simulink library "MBDS_Subsystems"  (R2018b)
settings: Solver=ode45  StartTime=0.0  StopTime=10.0  RelTol=1e-3
libraries: KIBES_Signal x1429, MBDS_Modules x44, simulink x2
(part 3 of 15)

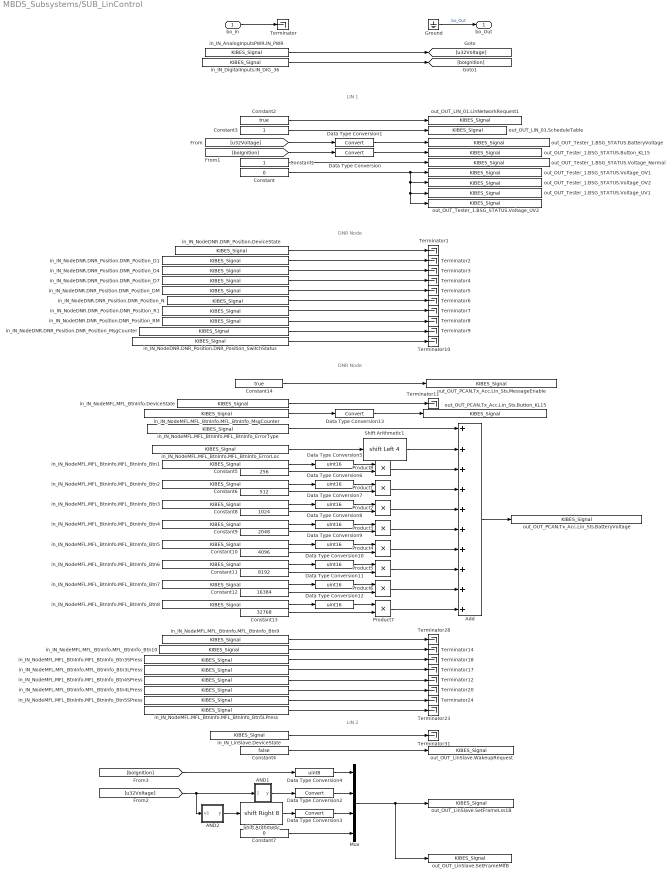
== system MBDS_Subsystems/SUB_LinControl ==
  note: LIN 2
  note: DNR Node
  note: DNR Node
  note: LIN 1
  bo_In : Inport  OutDataTypeStr=boolean
  AND1 : Subsystem  InitFcn=|  mask(AND){MBDS_LibraryBlock=on, BitwiseMode=on, Inputs=1, UseBitMask=on, BitMask='FF', OutDataTypeStr=Inherit: Inherit via back propagation, MBDS_BlockVersion=08.20.02}
      | if(exist('MBDS_BlockCallback', 'file'))
      |    MBDS_BlockCallback('Update', gcb);
      | end
      mask prompts: MBDS_LibraryBlock "MBDS library block"; BitwiseMode "Use 'bitwise' mode"; Inputs "Number of input ports:"; UseBitMask "Use bit mask"; BitMask "Bit mask:"; OutDataTypeStr "Output data type:"; MBDS_BlockVersion "Version:"
      mask help: Logical or bitwise AND operator. For multiple inputs, operators are applied across the inputs. For a single input, operators are applied across the input vector. In bitwise mode a bit mask can be applied onto single input signals.
      mask init: same as MBDS_Subsystems/SUB_DateTime/AND
      settings: AttributesFormatString=bitwise
      mask Help: eval(['open([workdir(''library_dir:''),''\Blockset\help\'',get_param(gcb,''MaskType''),''.html''])'])
      mask Callback BitwiseMode:
      | if(exist('MBDS_BlockCallback', 'file'))
      |    MBDS_BlockCallback('BitwiseMode', gcb);
      | end
      mask Callback Inputs:
      | if(exist('MBDS_BlockCallback', 'file'))
      |    MBDS_BlockCallback('Inputs', gcb);
      | end
      mask Callback UseBitMask:
      | if(exist('MBDS_BlockCallback', 'file'))
      |    MBDS_BlockCallback('UseBitMask', gcb);
      | end
      mask Callback BitMask:
      | if(exist('MBDS_BlockCallback', 'file'))
      |    MBDS_BlockCallback('BitMask', gcb);
      | end
      mask TypeOptions OutDataTypeStr: Inherit: Inherit via back propagation | int8 | uint8 | int16 | uint16 | int32 | uint32 | boolean
      mask Callback OutDataTypeStr:
      | % Adopt Value
      | if(exist('MBDS_BlockCallback', 'file'))
      |    MBDS_BlockCallback('OutDataTypeStr', gcb);
      | end
      mask DialogControl ParameterTabVar0 Prompt: Main
      mask DialogControl ParameterTabVar01 Prompt: Signal Attributes
      mask DialogControl ParameterTabVar012 Prompt: Version
      mask Display:
      | % Show icon or block text
      | if(UseBitMask)
      |    if(isnumeric(BitMask))
      |       BitMaskString = ['0x',dec2hex(floor(BitMask))];
      |    elseif(ischar(BitMask))
      |       BitMaskString = ['0x',upper(BitMask)];
      |    else
      |       BitMaskString = '???';
      |    end
      |    disp(sprintf(['AND\n', BitMaskString]))
      | else
      |    disp('AND')
      | end
  AND2 : Subsystem  InitFcn=|  mask(AND){MBDS_LibraryBlock=on, BitwiseMode=on, Inputs=1, UseBitMask=on, BitMask='FF00', OutDataTypeStr=Inherit: Inherit via back propagation, MBDS_BlockVersion=08.20.02}
      | if(exist('MBDS_BlockCallback', 'file'))
      |    MBDS_BlockCallback('Update', gcb);
      | end
      mask prompts: MBDS_LibraryBlock "MBDS library block"; BitwiseMode "Use 'bitwise' mode"; Inputs "Number of input ports:"; UseBitMask "Use bit mask"; BitMask "Bit mask:"; OutDataTypeStr "Output data type:"; MBDS_BlockVersion "Version:"
      mask help: Logical or bitwise AND operator. For multiple inputs, operators are applied across the inputs. For a single input, operators are applied across the input vector. In bitwise mode a bit mask can be applied onto single input signals.
      mask init: same as MBDS_Subsystems/SUB_DateTime/AND
      settings: AttributesFormatString=bitwise
      mask Help: eval(['open([workdir(''library_dir:''),''\Blockset\help\'',get_param(gcb,''MaskType''),''.html''])'])
      mask Callback BitwiseMode:
      | if(exist('MBDS_BlockCallback', 'file'))
      |    MBDS_BlockCallback('BitwiseMode', gcb);
      | end
      mask Callback Inputs:
      | if(exist('MBDS_BlockCallback', 'file'))
      |    MBDS_BlockCallback('Inputs', gcb);
      | end
      mask Callback UseBitMask:
      | if(exist('MBDS_BlockCallback', 'file'))
      |    MBDS_BlockCallback('UseBitMask', gcb);
      | end
      mask Callback BitMask:
      | if(exist('MBDS_BlockCallback', 'file'))
      |    MBDS_BlockCallback('BitMask', gcb);
      | end
      mask TypeOptions OutDataTypeStr: Inherit: Inherit via back propagation | int8 | uint8 | int16 | uint16 | int32 | uint32 | boolean
      mask Callback OutDataTypeStr:
      | % Adopt Value
      | if(exist('MBDS_BlockCallback', 'file'))
      |    MBDS_BlockCallback('OutDataTypeStr', gcb);
      | end
      mask DialogControl ParameterTabVar0 Prompt: Main
      mask DialogControl ParameterTabVar01 Prompt: Signal Attributes
      mask DialogControl ParameterTabVar012 Prompt: Version
      mask Display:
      | % Show icon or block text
      | if(UseBitMask)
      |    if(isnumeric(BitMask))
      |       BitMaskString = ['0x',dec2hex(floor(BitMask))];
      |    elseif(ischar(BitMask))
      |       BitMaskString = ['0x',upper(BitMask)];
      |    else
      |       BitMaskString = '???';
      |    end
      |    disp(sprintf(['AND\n', BitMaskString]))
      | else
      |    disp('AND')
      | end
  Add : Sum  InitFcn=|  Inputs=++++++++++  AccumDataTypeStr=uint16  OutDataTypeStr=uint16  SaturateOnIntegerOverflow=on
      | if(exist('MBDS_BlockCallback', 'file'))
      |    MBDS_BlockCallback('Update', gcb);  
      | end
      settings: AttributesFormatString=Saturate: %<SaturateOnIntegerOverflow>
  Constant : Constant  InitFcn=|  Value=0  OutDataTypeStr=uint8
      | if(exist('MBDS_BlockCallback', 'file'))
      |    MBDS_BlockCallback('Update', gcb);  
      | end
  Constant1 : Constant  InitFcn=|  OutDataTypeStr=uint8
      | if(exist('MBDS_BlockCallback', 'file'))
      |    MBDS_BlockCallback('Update', gcb);  
      | end
  Constant10 : Constant  InitFcn=|  Value=4096  OutDataTypeStr=uint16
      | if(exist('MBDS_BlockCallback', 'file'))
      |    MBDS_BlockCallback('Update', gcb);  
      | end
  Constant11 : Constant  InitFcn=|  Value=8192  OutDataTypeStr=uint16
      | if(exist('MBDS_BlockCallback', 'file'))
      |    MBDS_BlockCallback('Update', gcb);  
      | end
  Constant12 : Constant  InitFcn=|  Value=16384  OutDataTypeStr=uint16
      | if(exist('MBDS_BlockCallback', 'file'))
      |    MBDS_BlockCallback('Update', gcb);  
      | end
  Constant13 : Constant  InitFcn=|  Value=32768  OutDataTypeStr=uint16
      | if(exist('MBDS_BlockCallback', 'file'))
      |    MBDS_BlockCallback('Update', gcb);  
      | end
  Constant14 : Constant  InitFcn=|  Value=true  OutDataTypeStr=boolean  LockScale=on
      | if(exist('MBDS_BlockCallback', 'file'))
      |    MBDS_BlockCallback('Update', gcb);  
      | end
  Constant2 : Constant  InitFcn=|  Value=true  OutDataTypeStr=boolean
      | if(exist('MBDS_BlockCallback', 'file'))
      |    MBDS_BlockCallback('Update', gcb);  
      | end
  Constant3 : Constant  InitFcn=|  OutDataTypeStr=uint8
      | if(exist('MBDS_BlockCallback', 'file'))
      |    MBDS_BlockCallback('Update', gcb);  
      | end
  Constant4 : Constant  InitFcn=|  Value=false  OutDataTypeStr=boolean
      | if(exist('MBDS_BlockCallback', 'file'))
      |    MBDS_BlockCallback('Update', gcb);  
      | end
  Constant5 : Constant  InitFcn=|  Value=256  OutDataTypeStr=uint16
      | if(exist('MBDS_BlockCallback', 'file'))
      |    MBDS_BlockCallback('Update', gcb);  
      | end
  Constant6 : Constant  InitFcn=|  Value=512  OutDataTypeStr=uint16
      | if(exist('MBDS_BlockCallback', 'file'))
      |    MBDS_BlockCallback('Update', gcb);  
      | end
  Constant7 : Constant  InitFcn=|  Value=0  OutDataTypeStr=uint8
      | if(exist('MBDS_BlockCallback', 'file'))
      |    MBDS_BlockCallback('Update', gcb);  
      | end
  Constant8 : Constant  InitFcn=|  Value=1024  OutDataTypeStr=uint16
      | if(exist('MBDS_BlockCallback', 'file'))
      |    MBDS_BlockCallback('Update', gcb);  
      | end
  Constant9 : Constant  InitFcn=|  Value=2048  OutDataTypeStr=uint16
      | if(exist('MBDS_BlockCallback', 'file'))
      |    MBDS_BlockCallback('Update', gcb);  
      | end
  Data Type Conversion : DataTypeConversion  InitFcn=|  SaturateOnIntegerOverflow=on
      | try
      |    MBDS_BlockCallback('Update', gcb);
      | end
      settings: AttributesFormatString=Saturate: %<SaturateOnIntegerOverflow>
  Data Type Conversion1 : DataTypeConversion  InitFcn=|  SaturateOnIntegerOverflow=on
      | try
      |    MBDS_BlockCallback('Update', gcb);
      | end
      settings: AttributesFormatString=Saturate: %<SaturateOnIntegerOverflow>
  Data Type Conversion10 : DataTypeConversion  InitFcn=|  OutDataTypeStr=uint16  SaturateOnIntegerOverflow=on
      | try
      |    MBDS_BlockCallback('Update', gcb);
      | end
      settings: AttributesFormatString=Saturate: %<SaturateOnIntegerOverflow>
  Data Type Conversion11 : DataTypeConversion  InitFcn=|  OutDataTypeStr=uint16  SaturateOnIntegerOverflow=on
      | try
      |    MBDS_BlockCallback('Update', gcb);
      | end
      settings: AttributesFormatString=Saturate: %<SaturateOnIntegerOverflow>
  Data Type Conversion12 : DataTypeConversion  InitFcn=|  OutDataTypeStr=uint16  SaturateOnIntegerOverflow=on
      | try
      |    MBDS_BlockCallback('Update', gcb);
      | end
      settings: AttributesFormatString=Saturate: %<SaturateOnIntegerOverflow>
  Data Type Conversion13 : DataTypeConversion  InitFcn=|  SaturateOnIntegerOverflow=on
      | try
      |    MBDS_BlockCallback('Update', gcb);
      | end
      settings: AttributesFormatString=Saturate: %<SaturateOnIntegerOverflow>
  Data Type Conversion2 : DataTypeConversion  InitFcn=|
      | try
      |    MBDS_BlockCallback('Update', gcb);
      | end
      settings: AttributesFormatString=Saturate: %<SaturateOnIntegerOverflow>
  Data Type Conversion3 : DataTypeConversion  InitFcn=|
      | try
      |    MBDS_BlockCallback('Update', gcb);
      | end
      settings: AttributesFormatString=Saturate: %<SaturateOnIntegerOverflow>
  Data Type Conversion4 : DataTypeConversion  InitFcn=|  OutDataTypeStr=uint8  SaturateOnIntegerOverflow=on
      | try
      |    MBDS_BlockCallback('Update', gcb);
      | end
      settings: AttributesFormatString=Saturate: %<SaturateOnIntegerOverflow>
  Data Type Conversion5 : DataTypeConversion  InitFcn=|  OutDataTypeStr=uint16  SaturateOnIntegerOverflow=on
      | try
      |    MBDS_BlockCallback('Update', gcb);
      | end
      settings: AttributesFormatString=Saturate: %<SaturateOnIntegerOverflow>
  Data Type Conversion6 : DataTypeConversion  InitFcn=|  OutDataTypeStr=uint16  SaturateOnIntegerOverflow=on
      | try
      |    MBDS_BlockCallback('Update', gcb);
      | end
      settings: AttributesFormatString=Saturate: %<SaturateOnIntegerOverflow>
  Data Type Conversion7 : DataTypeConversion  InitFcn=|  OutDataTypeStr=uint16  SaturateOnIntegerOverflow=on
      | try
      |    MBDS_BlockCallback('Update', gcb);
      | end
      settings: AttributesFormatString=Saturate: %<SaturateOnIntegerOverflow>
  Data Type Conversion8 : DataTypeConversion  InitFcn=|  OutDataTypeStr=uint16  SaturateOnIntegerOverflow=on
      | try
      |    MBDS_BlockCallback('Update', gcb);
      | end
      settings: AttributesFormatString=Saturate: %<SaturateOnIntegerOverflow>
  Data Type Conversion9 : DataTypeConversion  InitFcn=|  OutDataTypeStr=uint16  SaturateOnIntegerOverflow=on
      | try
      |    MBDS_BlockCallback('Update', gcb);
      | end
      settings: AttributesFormatString=Saturate: %<SaturateOnIntegerOverflow>
  Ground : Ground  InitFcn=|
      | try
      |    MBDS_BlockCallback('Update', gcb);
      | end
      settings: MoveFcn=UpdateBlockSize(gcb);
  Mux : Mux  InitFcn=|
      | try
      |    MBDS_BlockCallback('Update', gcb);
      | end
  Product1 : Product  InitFcn=|  Inputs=**  OutDataTypeStr=uint16  SaturateOnIntegerOverflow=on
      | if(exist('MBDS_BlockCallback', 'file'))
      |    MBDS_BlockCallback('Update', gcb);  
      | end
      settings: AttributesFormatString=Saturate: %<SaturateOnIntegerOverflow>
  Product2 : Product  InitFcn=|  Inputs=**  OutDataTypeStr=uint16  SaturateOnIntegerOverflow=on
      | if(exist('MBDS_BlockCallback', 'file'))
      |    MBDS_BlockCallback('Update', gcb);  
      | end
      settings: AttributesFormatString=Saturate: %<SaturateOnIntegerOverflow>
  Product3 : Product  InitFcn=|  Inputs=**  OutDataTypeStr=uint16  SaturateOnIntegerOverflow=on
      | if(exist('MBDS_BlockCallback', 'file'))
      |    MBDS_BlockCallback('Update', gcb);  
      | end
      settings: AttributesFormatString=Saturate: %<SaturateOnIntegerOverflow>
  Product4 : Product  InitFcn=|  Inputs=**  OutDataTypeStr=uint16  SaturateOnIntegerOverflow=on
      | if(exist('MBDS_BlockCallback', 'file'))
      |    MBDS_BlockCallback('Update', gcb);  
      | end
      settings: AttributesFormatString=Saturate: %<SaturateOnIntegerOverflow>
  Product5 : Product  InitFcn=|  Inputs=**  OutDataTypeStr=uint16  SaturateOnIntegerOverflow=on
      | if(exist('MBDS_BlockCallback', 'file'))
      |    MBDS_BlockCallback('Update', gcb);  
      | end
      settings: AttributesFormatString=Saturate: %<SaturateOnIntegerOverflow>
  Product6 : Product  InitFcn=|  Inputs=**  OutDataTypeStr=uint16  SaturateOnIntegerOverflow=on
      | if(exist('MBDS_BlockCallback', 'file'))
      |    MBDS_BlockCallback('Update', gcb);  
      | end
      settings: AttributesFormatString=Saturate: %<SaturateOnIntegerOverflow>
  Product7 : Product  InitFcn=|  Inputs=**  OutDataTypeStr=uint16  SaturateOnIntegerOverflow=on
      | if(exist('MBDS_BlockCallback', 'file'))
      |    MBDS_BlockCallback('Update', gcb);  
      | end
      settings: AttributesFormatString=Saturate: %<SaturateOnIntegerOverflow>
  Product8 : Product  InitFcn=|  Inputs=**  OutDataTypeStr=uint16  SaturateOnIntegerOverflow=on
      | if(exist('MBDS_BlockCallback', 'file'))
      |    MBDS_BlockCallback('Update', gcb);  
      | end
      settings: AttributesFormatString=Saturate: %<SaturateOnIntegerOverflow>
  Shift Arithmetic : ArithShift  InitFcn=|  BitShiftNumber=8  BitShiftDirection=Right
      | try
      |    MBDS_BlockCallback('Update', gcb);
      | end
  Shift Arithmetic1 : ArithShift  InitFcn=|  BitShiftNumber=4  BitShiftDirection=Left
      | try
      |    MBDS_BlockCallback('Update', gcb);
      | end
  Terminator{,1..12,14,17..18,20,23..24,28,31} (21 alike) : Terminator
      settings: MoveFcn=UpdateBlockSize(gcb);
      settings: InitFcn=|
      | try
      |    MBDS_BlockCallback('Update', gcb);
      | end
  in_IN_AnalogInputsPWR.IN_PWR : KIBES_Signal/KIBES_Signal  MBDS_LibraryBlock=on  DatabaseKey=721  SignalName=IN_AnalogInputsPWR.IN_PWR  SymbolName=IN_AnalogInputsPWR_IN_PWR_000721  DataType=uint32  Init=0  Slope=1  Bias=0  DataSize=1  fpDataType=uint32  BlockIOType=Inport  DeviceType=0
  in_IN_DigitalInputs.IN_DIG_36 : KIBES_Signal/KIBES_Signal  MBDS_LibraryBlock=on  DatabaseKey=60  SignalName=IN_DigitalInputs.IN_DIG_36  SymbolName=IN_DigitalInputs_IN_DIG_36_000060  DataType=boolean  Init=0  Slope=1  Bias=0  DataSize=1  fpDataType=boolean  BlockIOType=Inport  DeviceType=0
  in_IN_LinSlave.DeviceState : KIBES_Signal/KIBES_Signal  MBDS_LibraryBlock=on  DatabaseKey=2325  SignalName=IN_LinSlave.DeviceState  SymbolName=IN_LinSlave_DeviceState_002325  DataType=uint16  Init=0  Slope=1  Bias=0  DataSize=1  fpDataType=uint16  BlockIOType=Inport  DeviceType=0
  in_IN_NodeDNR.DNR_Position.DNR_Position_D1 : KIBES_Signal/KIBES_Signal  MBDS_LibraryBlock=on  DatabaseKey=1352  SignalName=IN_NodeDNR.DNR_Position.DNR_Position_D1  SymbolName=IN_NodeDNR_DNR_Position_DNR_Position_D1_001352  DataType=uint8  Init=0  Slope=1  Bias=0  DataSize=1  fpDataType=uint8  BlockIOType=Inport  DeviceType=0
  in_IN_NodeDNR.DNR_Position.DNR_Position_D4 : KIBES_Signal/KIBES_Signal  MBDS_LibraryBlock=on  DatabaseKey=1353  SignalName=IN_NodeDNR.DNR_Position.DNR_Position_D4  SymbolName=IN_NodeDNR_DNR_Position_DNR_Position_D4_001353  DataType=uint8  Init=0  Slope=1  Bias=0  DataSize=1  fpDataType=uint8  BlockIOType=Inport  DeviceType=0
  in_IN_NodeDNR.DNR_Position.DNR_Position_D7 : KIBES_Signal/KIBES_Signal  MBDS_LibraryBlock=on  DatabaseKey=1354  SignalName=IN_NodeDNR.DNR_Position.DNR_Position_D7  SymbolName=IN_NodeDNR_DNR_Position_DNR_Position_D7_001354  DataType=uint8  Init=0  Slope=1  Bias=0  DataSize=1  fpDataType=uint8  BlockIOType=Inport  DeviceType=0
  in_IN_NodeDNR.DNR_Position.DNR_Position_DM : KIBES_Signal/KIBES_Signal  MBDS_LibraryBlock=on  DatabaseKey=1355  SignalName=IN_NodeDNR.DNR_Position.DNR_Position_DM  SymbolName=IN_NodeDNR_DNR_Position_DNR_Position_DM_001355  DataType=uint8  Init=0  Slope=1  Bias=0  DataSize=1  fpDataType=uint8  BlockIOType=Inport  DeviceType=0
  in_IN_NodeDNR.DNR_Position.DNR_Position_MsgCounter : KIBES_Signal/KIBES_Signal  MBDS_LibraryBlock=on  DatabaseKey=1356  SignalName=IN_NodeDNR.DNR_Position.DNR_Position_MsgCounter  SymbolName=IN_NodeDNR_DNR_Position_DNR_Position_MsgCounter_001356  DataType=uint8  Init=0  Slope=1  Bias=0  DataSize=1  fpDataType=uint8  BlockIOType=Inport  DeviceType=0
  in_IN_NodeDNR.DNR_Position.DNR_Position_N : KIBES_Signal/KIBES_Signal  MBDS_LibraryBlock=on  DatabaseKey=1351  SignalName=IN_NodeDNR.DNR_Position.DNR_Position_N  SymbolName=IN_NodeDNR_DNR_Position_DNR_Position_N_001351  DataType=uint8  Init=0  Slope=1  Bias=0  DataSize=1  fpDataType=uint8  BlockIOType=Inport  DeviceType=0
  in_IN_NodeDNR.DNR_Position.DNR_Position_R1 : KIBES_Signal/KIBES_Signal  MBDS_LibraryBlock=on  DatabaseKey=1350  SignalName=IN_NodeDNR.DNR_Position.DNR_Position_R1  SymbolName=IN_NodeDNR_DNR_Position_DNR_Position_R1_001350  DataType=uint8  Init=0  Slope=1  Bias=0  DataSize=1  fpDataType=uint8  BlockIOType=Inport  DeviceType=0
  in_IN_NodeDNR.DNR_Position.DNR_Position_RM : KIBES_Signal/KIBES_Signal  MBDS_LibraryBlock=on  DatabaseKey=1349  SignalName=IN_NodeDNR.DNR_Position.DNR_Position_RM  SymbolName=IN_NodeDNR_DNR_Position_DNR_Position_RM_001349  DataType=uint8  Init=0  Slope=1  Bias=0  DataSize=1  fpDataType=uint8  BlockIOType=Inport  DeviceType=0
  in_IN_NodeDNR.DNR_Position.DNR_Position_SwitchStatus : KIBES_Signal/KIBES_Signal  MBDS_LibraryBlock=on  DatabaseKey=1357  SignalName=IN_NodeDNR.DNR_Position.DNR_Position_SwitchStatus  SymbolName=IN_NodeDNR_DNR_Position_DNR_Position_SwitchStatus_001357  DataType=uint8  Init=0  Slope=1  Bias=0  DataSize=1  fpDataType=uint8  BlockIOType=Inport  DeviceType=0
  in_IN_NodeDNR.DNR_Position.DeviceState : KIBES_Signal/KIBES_Signal  MBDS_LibraryBlock=on  DatabaseKey=2273  SignalName=IN_NodeDNR.DNR_Position.DeviceState  SymbolName=IN_NodeDNR_DNR_Position_DeviceState_002273  DataType=uint16  Init=0  Slope=1  Bias=0  DataSize=1  fpDataType=uint16  BlockIOType=Inport  DeviceType=0
  in_IN_NodeMFL.MFL_BtnInfo.DeviceState : KIBES_Signal/KIBES_Signal  MBDS_LibraryBlock=on  DatabaseKey=2272  SignalName=IN_NodeMFL.MFL_BtnInfo.DeviceState  SymbolName=IN_NodeMFL_MFL_BtnInfo_DeviceState_002272  DataType=uint16  Init=0  Slope=1  Bias=0  DataSize=1  fpDataType=uint16  BlockIOType=Inport  DeviceType=0
  in_IN_NodeMFL.MFL_BtnInfo.MFL_BtnInfo_Btn1 : KIBES_Signal/KIBES_Signal  MBDS_LibraryBlock=on  DatabaseKey=1361  SignalName=IN_NodeMFL.MFL_BtnInfo.MFL_BtnInfo_Btn1  SymbolName=IN_NodeMFL_MFL_BtnInfo_MFL_BtnInfo_Btn1_001361  DataType=uint8  Init=0  Slope=1  Bias=0  DataSize=1  fpDataType=uint8  BlockIOType=Inport  DeviceType=0
  in_IN_NodeMFL.MFL_BtnInfo.MFL_BtnInfo_Btn10 : KIBES_Signal/KIBES_Signal  MBDS_LibraryBlock=on  DatabaseKey=1370  SignalName=IN_NodeMFL.MFL_BtnInfo.MFL_BtnInfo_Btn10  SymbolName=IN_NodeMFL_MFL_BtnInfo_MFL_BtnInfo_Btn10_001370  DataType=uint8  Init=0  Slope=1  Bias=0  DataSize=1  fpDataType=uint8  BlockIOType=Inport  DeviceType=0
  in_IN_NodeMFL.MFL_BtnInfo.MFL_BtnInfo_Btn2 : KIBES_Signal/KIBES_Signal  MBDS_LibraryBlock=on  DatabaseKey=1362  SignalName=IN_NodeMFL.MFL_BtnInfo.MFL_BtnInfo_Btn2  SymbolName=IN_NodeMFL_MFL_BtnInfo_MFL_BtnInfo_Btn2_001362  DataType=uint8  Init=0  Slope=1  Bias=0  DataSize=1  fpDataType=uint8  BlockIOType=Inport  DeviceType=0
  in_IN_NodeMFL.MFL_BtnInfo.MFL_BtnInfo_Btn3 : KIBES_Signal/KIBES_Signal  MBDS_LibraryBlock=on  DatabaseKey=1363  SignalName=IN_NodeMFL.MFL_BtnInfo.MFL_BtnInfo_Btn3  SymbolName=IN_NodeMFL_MFL_BtnInfo_MFL_BtnInfo_Btn3_001363  DataType=uint8  Init=0  Slope=1  Bias=0  DataSize=1  fpDataType=uint8  BlockIOType=Inport  DeviceType=0
  in_IN_NodeMFL.MFL_BtnInfo.MFL_BtnInfo_Btn3LPress : KIBES_Signal/KIBES_Signal  MBDS_LibraryBlock=on  DatabaseKey=1372  SignalName=IN_NodeMFL.MFL_BtnInfo.MFL_BtnInfo_Btn3LPress  SymbolName=IN_NodeMFL_MFL_BtnInfo_MFL_BtnInfo_Btn3LPress_001372  DataType=uint8  Init=0  Slope=1  Bias=0  DataSize=1  fpDataType=uint8  BlockIOType=Inport  DeviceType=0
  in_IN_NodeMFL.MFL_BtnInfo.MFL_BtnInfo_Btn3SPress : KIBES_Signal/KIBES_Signal  MBDS_LibraryBlock=on  DatabaseKey=1371  SignalName=IN_NodeMFL.MFL_BtnInfo.MFL_BtnInfo_Btn3SPress  SymbolName=IN_NodeMFL_MFL_BtnInfo_MFL_BtnInfo_Btn3SPress_001371  DataType=uint8  Init=0  Slope=1  Bias=0  DataSize=1  fpDataType=uint8  BlockIOType=Inport  DeviceType=0
  in_IN_NodeMFL.MFL_BtnInfo.MFL_BtnInfo_Btn4 : KIBES_Signal/KIBES_Signal  MBDS_LibraryBlock=on  DatabaseKey=1364  SignalName=IN_NodeMFL.MFL_BtnInfo.MFL_BtnInfo_Btn4  SymbolName=IN_NodeMFL_MFL_BtnInfo_MFL_BtnInfo_Btn4_001364  DataType=uint8  Init=0  Slope=1  Bias=0  DataSize=1  fpDataType=uint8  BlockIOType=Inport  DeviceType=0
  in_IN_NodeMFL.MFL_BtnInfo.MFL_BtnInfo_Btn4LPress : KIBES_Signal/KIBES_Signal  MBDS_LibraryBlock=on  DatabaseKey=1374  SignalName=IN_NodeMFL.MFL_BtnInfo.MFL_BtnInfo_Btn4LPress  SymbolName=IN_NodeMFL_MFL_BtnInfo_MFL_BtnInfo_Btn4LPress_001374  DataType=uint8  Init=0  Slope=1  Bias=0  DataSize=1  fpDataType=uint8  BlockIOType=Inport  DeviceType=0
  in_IN_NodeMFL.MFL_BtnInfo.MFL_BtnInfo_Btn4SPress : KIBES_Signal/KIBES_Signal  MBDS_LibraryBlock=on  DatabaseKey=1373  SignalName=IN_NodeMFL.MFL_BtnInfo.MFL_BtnInfo_Btn4SPress  SymbolName=IN_NodeMFL_MFL_BtnInfo_MFL_BtnInfo_Btn4SPress_001373  DataType=uint8  Init=0  Slope=1  Bias=0  DataSize=1  fpDataType=uint8  BlockIOType=Inport  DeviceType=0
  in_IN_NodeMFL.MFL_BtnInfo.MFL_BtnInfo_Btn5 : KIBES_Signal/KIBES_Signal  MBDS_LibraryBlock=on  DatabaseKey=1365  SignalName=IN_NodeMFL.MFL_BtnInfo.MFL_BtnInfo_Btn5  SymbolName=IN_NodeMFL_MFL_BtnInfo_MFL_BtnInfo_Btn5_001365  DataType=uint8  Init=0  Slope=1  Bias=0  DataSize=1  fpDataType=uint8  BlockIOType=Inport  DeviceType=0
  in_IN_NodeMFL.MFL_BtnInfo.MFL_BtnInfo_Btn5LPress : KIBES_Signal/KIBES_Signal  MBDS_LibraryBlock=on  DatabaseKey=1376  SignalName=IN_NodeMFL.MFL_BtnInfo.MFL_BtnInfo_Btn5LPress  SymbolName=IN_NodeMFL_MFL_BtnInfo_MFL_BtnInfo_Btn5LPress_001376  DataType=uint8  Init=0  Slope=1  Bias=0  DataSize=1  fpDataType=uint8  BlockIOType=Inport  DeviceType=0
  in_IN_NodeMFL.MFL_BtnInfo.MFL_BtnInfo_Btn5SPress : KIBES_Signal/KIBES_Signal  MBDS_LibraryBlock=on  DatabaseKey=1375  SignalName=IN_NodeMFL.MFL_BtnInfo.MFL_BtnInfo_Btn5SPress  SymbolName=IN_NodeMFL_MFL_BtnInfo_MFL_BtnInfo_Btn5SPress_001375  DataType=uint8  Init=0  Slope=1  Bias=0  DataSize=1  fpDataType=uint8  BlockIOType=Inport  DeviceType=0
  in_IN_NodeMFL.MFL_BtnInfo.MFL_BtnInfo_Btn6 : KIBES_Signal/KIBES_Signal  MBDS_LibraryBlock=on  DatabaseKey=1366  SignalName=IN_NodeMFL.MFL_BtnInfo.MFL_BtnInfo_Btn6  SymbolName=IN_NodeMFL_MFL_BtnInfo_MFL_BtnInfo_Btn6_001366  DataType=uint8  Init=0  Slope=1  Bias=0  DataSize=1  fpDataType=uint8  BlockIOType=Inport  DeviceType=0
  in_IN_NodeMFL.MFL_BtnInfo.MFL_BtnInfo_Btn7 : KIBES_Signal/KIBES_Signal  MBDS_LibraryBlock=on  DatabaseKey=1367  SignalName=IN_NodeMFL.MFL_BtnInfo.MFL_BtnInfo_Btn7  SymbolName=IN_NodeMFL_MFL_BtnInfo_MFL_BtnInfo_Btn7_001367  DataType=uint8  Init=0  Slope=1  Bias=0  DataSize=1  fpDataType=uint8  BlockIOType=Inport  DeviceType=0
  in_IN_NodeMFL.MFL_BtnInfo.MFL_BtnInfo_Btn8 : KIBES_Signal/KIBES_Signal  MBDS_LibraryBlock=on  DatabaseKey=1368  SignalName=IN_NodeMFL.MFL_BtnInfo.MFL_BtnInfo_Btn8  SymbolName=IN_NodeMFL_MFL_BtnInfo_MFL_BtnInfo_Btn8_001368  DataType=uint8  Init=0  Slope=1  Bias=0  DataSize=1  fpDataType=uint8  BlockIOType=Inport  DeviceType=0
  in_IN_NodeMFL.MFL_BtnInfo.MFL_BtnInfo_Btn9 : KIBES_Signal/KIBES_Signal  MBDS_LibraryBlock=on  DatabaseKey=1369  SignalName=IN_NodeMFL.MFL_BtnInfo.MFL_BtnInfo_Btn9  SymbolName=IN_NodeMFL_MFL_BtnInfo_MFL_BtnInfo_Btn9_001369  DataType=uint8  Init=0  Slope=1  Bias=0  DataSize=1  fpDataType=uint8  BlockIOType=Inport  DeviceType=0
  in_IN_NodeMFL.MFL_BtnInfo.MFL_BtnInfo_ErrorLoc : KIBES_Signal/KIBES_Signal  MBDS_LibraryBlock=on  DatabaseKey=1360  SignalName=IN_NodeMFL.MFL_BtnInfo.MFL_BtnInfo_ErrorLoc  SymbolName=IN_NodeMFL_MFL_BtnInfo_MFL_BtnInfo_ErrorLoc_001360  DataType=uint8  Init=0  Slope=1  Bias=0  DataSize=1  fpDataType=uint8  BlockIOType=Inport  DeviceType=0
  in_IN_NodeMFL.MFL_BtnInfo.MFL_BtnInfo_ErrorType : KIBES_Signal/KIBES_Signal  MBDS_LibraryBlock=on  DatabaseKey=1359  SignalName=IN_NodeMFL.MFL_BtnInfo.MFL_BtnInfo_ErrorType  SymbolName=IN_NodeMFL_MFL_BtnInfo_MFL_BtnInfo_ErrorType_001359  DataType=uint8  Init=0  Slope=1  Bias=0  DataSize=1  fpDataType=uint8  BlockIOType=Inport  DeviceType=0
  in_IN_NodeMFL.MFL_BtnInfo.MFL_BtnInfo_MsgCounter : KIBES_Signal/KIBES_Signal  MBDS_LibraryBlock=on  DatabaseKey=1358  SignalName=IN_NodeMFL.MFL_BtnInfo.MFL_BtnInfo_MsgCounter  SymbolName=IN_NodeMFL_MFL_BtnInfo_MFL_BtnInfo_MsgCounter_001358  DataType=uint8  Init=0  Slope=1  Bias=0  DataSize=1  fpDataType=uint8  BlockIOType=Inport  DeviceType=0
  out_OUT_LIN_01.LinNetworkRequest1 : KIBES_Signal/KIBES_Signal  MBDS_LibraryBlock=on  DatabaseKey=1396  SignalName=OUT_LIN_01.LinNetworkRequest1  SymbolName=OUT_LIN_01_LinNetworkRequest1_001396  DataType=boolean  Init=0  Slope=1  Bias=0  DataSize=1  fpDataType=boolean  BlockIOType=Outport  DeviceType=0
  out_OUT_LIN_01.ScheduleTable : KIBES_Signal/KIBES_Signal  MBDS_LibraryBlock=on  DatabaseKey=1397  SignalName=OUT_LIN_01.ScheduleTable  SymbolName=OUT_LIN_01_ScheduleTable_001397  DataType=uint8  Init=0  Slope=1  Bias=0  DataSize=1  fpDataType=uint8  BlockIOType=Outport  DeviceType=0
  out_OUT_LinSlave.SetFrameLss1B : KIBES_Signal/KIBES_Signal  MBDS_LibraryBlock=on  DatabaseKey=2326  SignalName=OUT_LinSlave.SetFrameLss1B  SymbolName=OUT_LinSlave_SetFrameLss1B_002326  DataType=uint8  Init=[0 0 0 0]  Slope=1  Bias=0  DataSize=4  fpDataType=uint8  BlockIOType=Outport  DeviceType=0
  out_OUT_LinSlave.SetFrameMlfB : KIBES_Signal/KIBES_Signal  MBDS_LibraryBlock=on  DatabaseKey=2327  SignalName=OUT_LinSlave.SetFrameMlfB  SymbolName=OUT_LinSlave_SetFrameMlfB_002327  DataType=uint8  Init=[0 0 0 0]  Slope=1  Bias=0  DataSize=4  fpDataType=uint8  BlockIOType=Outport  DeviceType=0
  out_OUT_LinSlave.WakeupRequest : KIBES_Signal/KIBES_Signal  MBDS_LibraryBlock=on  DatabaseKey=2328  SignalName=OUT_LinSlave.WakeupRequest  SymbolName=OUT_LinSlave_WakeupRequest_002328  DataType=boolean  Init=0  Slope=1  Bias=0  DataSize=1  fpDataType=boolean  BlockIOType=Outport  DeviceType=0
  out_OUT_PCAN.Tx_Acc.Lin_Sts.BatteryVoltage : KIBES_Signal/KIBES_Signal  MBDS_LibraryBlock=on  DatabaseKey=1647  SignalName=OUT_PCAN.Tx_Acc.Lin_Sts.BatteryVoltage  SymbolName=OUT_PCAN_Tx_Acc_Lin_Sts_BatteryVoltage_001647  DataType=uint16  Init=0  Slope=1  Bias=0  DataSize=1  fpDataType=uint16  BlockIOType=Outport  DeviceType=0
  out_OUT_PCAN.Tx_Acc.Lin_Sts.Button_KL15 : KIBES_Signal/KIBES_Signal  MBDS_LibraryBlock=on  DatabaseKey=1648  SignalName=OUT_PCAN.Tx_Acc.Lin_Sts.Button_KL15  SymbolName=OUT_PCAN_Tx_Acc_Lin_Sts_Button_KL15_001648  DataType=boolean  Init=0  Slope=1  Bias=0  DataSize=1  fpDataType=boolean  BlockIOType=Outport  DeviceType=0
  out_OUT_PCAN.Tx_Acc.Lin_Sts.MessageEnable : KIBES_Signal/KIBES_Signal  MBDS_LibraryBlock=on  DatabaseKey=1677  SignalName=OUT_PCAN.Tx_Acc.Lin_Sts.MessageEnable  SymbolName=OUT_PCAN_Tx_Acc_Lin_Sts_MessageEnable_001677  DataType=boolean  Init=0  Slope=1  Bias=0  DataSize=1  fpDataType=boolean  BlockIOType=Outport  DeviceType=0
  out_OUT_Tester_1.BSG_STATUS.BatteryVoltage : KIBES_Signal/KIBES_Signal  MBDS_LibraryBlock=on  DatabaseKey=1395  SignalName=OUT_Tester_1.BSG_STATUS.BatteryVoltage  SymbolName=OUT_Tester_1_BSG_STATUS_BatteryVoltage_001395  DataType=uint16  Init=0  Slope=1  Bias=0  DataSize=1  fpDataType=uint16  BlockIOType=Outport  DeviceType=0
  out_OUT_Tester_1.BSG_STATUS.Button_KL15 : KIBES_Signal/KIBES_Signal  MBDS_LibraryBlock=on  DatabaseKey=1389  SignalName=OUT_Tester_1.BSG_STATUS.Button_KL15  SymbolName=OUT_Tester_1_BSG_STATUS_Button_KL15_001389  DataType=uint8  Init=0  Slope=1  Bias=0  DataSize=1  fpDataType=uint8  BlockIOType=Outport  DeviceType=0
  out_OUT_Tester_1.BSG_STATUS.Voltage_Normal : KIBES_Signal/KIBES_Signal  MBDS_LibraryBlock=on  DatabaseKey=1390  SignalName=OUT_Tester_1.BSG_STATUS.Voltage_Normal  SymbolName=OUT_Tester_1_BSG_STATUS_Voltage_Normal_001390  DataType=uint8  Init=0  Slope=1  Bias=0  DataSize=1  fpDataType=uint8  BlockIOType=Outport  DeviceType=0
  out_OUT_Tester_1.BSG_STATUS.Voltage_OV1 : KIBES_Signal/KIBES_Signal  MBDS_LibraryBlock=on  DatabaseKey=1391  SignalName=OUT_Tester_1.BSG_STATUS.Voltage_OV1  SymbolName=OUT_Tester_1_BSG_STATUS_Voltage_OV1_001391  DataType=uint8  Init=0  Slope=1  Bias=0  DataSize=1  fpDataType=uint8  BlockIOType=Outport  DeviceType=0
  out_OUT_Tester_1.BSG_STATUS.Voltage_OV2 : KIBES_Signal/KIBES_Signal  MBDS_LibraryBlock=on  DatabaseKey=1392  SignalName=OUT_Tester_1.BSG_STATUS.Voltage_OV2  SymbolName=OUT_Tester_1_BSG_STATUS_Voltage_OV2_001392  DataType=uint8  Init=0  Slope=1  Bias=0  DataSize=1  fpDataType=uint8  BlockIOType=Outport  DeviceType=0
  out_OUT_Tester_1.BSG_STATUS.Voltage_UV1 : KIBES_Signal/KIBES_Signal  MBDS_LibraryBlock=on  DatabaseKey=1393  SignalName=OUT_Tester_1.BSG_STATUS.Voltage_UV1  SymbolName=OUT_Tester_1_BSG_STATUS_Voltage_UV1_001393  DataType=uint8  Init=0  Slope=1  Bias=0  DataSize=1  fpDataType=uint8  BlockIOType=Outport  DeviceType=0
  out_OUT_Tester_1.BSG_STATUS.Voltage_UV2 : KIBES_Signal/KIBES_Signal  MBDS_LibraryBlock=on  DatabaseKey=1394  SignalName=OUT_Tester_1.BSG_STATUS.Voltage_UV2  SymbolName=OUT_Tester_1_BSG_STATUS_Voltage_UV2_001394  DataType=uint8  Init=0  Slope=1  Bias=0  DataSize=1  fpDataType=uint8  BlockIOType=Outport  DeviceType=0
  bo_Out : Outport  OutDataTypeStr=boolean
  wires:
  Data Type Conversion13/1 -> out_OUT_PCAN.Tx_Acc.Lin_Sts.Button_KL15/1
  Constant14/1 -> out_OUT_PCAN.Tx_Acc.Lin_Sts.MessageEnable/1
  Add/1 -> out_OUT_PCAN.Tx_Acc.Lin_Sts.BatteryVoltage/1
  Constant13/1 -> Product7/2
  Constant12/1 -> Product6/2
  Constant11/1 -> Product5/2
  Constant10/1 -> Product4/2
  Constant9/1 -> Product3/2
  Constant8/1 -> Product2/2
  Constant6/1 -> Product1/2
  Constant5/1 -> Product8/2
  Data Type Conversion12/1 -> Product7/1
  Data Type Conversion11/1 -> Product6/1
  Data Type Conversion10/1 -> Product5/1
  Data Type Conversion9/1 -> Product4/1
  Data Type Conversion8/1 -> Product3/1
  Data Type Conversion7/1 -> Product2/1
  Data Type Conversion6/1 -> Product1/1
  Data Type Conversion5/1 -> Product8/1
  Product7/1 -> Add/10
  Product6/1 -> Add/9
  Product5/1 -> Add/8
  Product4/1 -> Add/7
  Product3/1 -> Add/6
  Product2/1 -> Add/5
  Product1/1 -> Add/4
  Product8/1 -> Add/3
  Shift Arithmetic1/1 -> Add/2
  [boIgnition] -> Data Type Conversion4/1
  Data Type Conversion4/1 -> Mux/1
  Shift Arithmetic/1 -> Data Type Conversion3/1
  AND2/1(y) -> Shift Arithmetic/1
  Data Type Conversion3/1 -> Mux/3
  [u32Voltage] -> AND1/1(u1), AND2/1(u1)
  AND1/1(y) -> Data Type Conversion2/1
  Data Type Conversion2/1 -> Mux/2
  in_IN_DigitalInputs.IN_DIG_36/1 -> [boIgnition]
  in_IN_AnalogInputsPWR.IN_PWR/1 -> [u32Voltage]
  Constant7/1 -> Mux/4
  Mux/1 -> out_OUT_LinSlave.SetFrameLss1B/1, out_OUT_LinSlave.SetFrameMlfB/1
  Constant4/1 -> out_OUT_LinSlave.WakeupRequest/1
  in_IN_LinSlave.DeviceState/1 -> Terminator31/1
  in_IN_NodeMFL.MFL_BtnInfo.MFL_BtnInfo_MsgCounter/1 -> Data Type Conversion13/1
  in_IN_NodeMFL.MFL_BtnInfo.MFL_BtnInfo_ErrorType/1 -> Add/1
  in_IN_NodeMFL.MFL_BtnInfo.MFL_BtnInfo_ErrorLoc/1 -> Shift Arithmetic1/1
  in_IN_NodeMFL.MFL_BtnInfo.MFL_BtnInfo_Btn9/1 -> Terminator28/1
  in_IN_NodeMFL.MFL_BtnInfo.MFL_BtnInfo_Btn8/1 -> Data Type Conversion12/1
  in_IN_NodeMFL.MFL_BtnInfo.MFL_BtnInfo_Btn7/1 -> Data Type Conversion11/1
  in_IN_NodeMFL.MFL_BtnInfo.MFL_BtnInfo_Btn6/1 -> Data Type Conversion10/1
  in_IN_NodeMFL.MFL_BtnInfo.MFL_BtnInfo_Btn5SPress/1 -> Terminator24/1
  in_IN_NodeMFL.MFL_BtnInfo.MFL_BtnInfo_Btn5LPress/1 -> Terminator23/1
  in_IN_NodeMFL.MFL_BtnInfo.MFL_BtnInfo_Btn5/1 -> Data Type Conversion9/1
  in_IN_NodeMFL.MFL_BtnInfo.MFL_BtnInfo_Btn4SPress/1 -> Terminator12/1
  in_IN_NodeMFL.MFL_BtnInfo.MFL_BtnInfo_Btn4LPress/1 -> Terminator20/1
  in_IN_NodeMFL.MFL_BtnInfo.MFL_BtnInfo_Btn4/1 -> Data Type Conversion8/1
  in_IN_NodeMFL.MFL_BtnInfo.MFL_BtnInfo_Btn3SPress/1 -> Terminator18/1
  in_IN_NodeMFL.MFL_BtnInfo.MFL_BtnInfo_Btn3LPress/1 -> Terminator17/1
  in_IN_NodeMFL.MFL_BtnInfo.MFL_BtnInfo_Btn3/1 -> Data Type Conversion7/1
  in_IN_NodeMFL.MFL_BtnInfo.MFL_BtnInfo_Btn2/1 -> Data Type Conversion6/1
  in_IN_NodeMFL.MFL_BtnInfo.MFL_BtnInfo_Btn10/1 -> Terminator14/1
  in_IN_NodeMFL.MFL_BtnInfo.MFL_BtnInfo_Btn1/1 -> Data Type Conversion5/1
  in_IN_NodeMFL.MFL_BtnInfo.DeviceState/1 -> Terminator11/1
  in_IN_NodeDNR.DNR_Position.DNR_Position_SwitchStatus/1 -> Terminator10/1
  in_IN_NodeDNR.DNR_Position.DNR_Position_MsgCounter/1 -> Terminator9/1
  in_IN_NodeDNR.DNR_Position.DNR_Position_RM/1 -> Terminator8/1
  in_IN_NodeDNR.DNR_Position.DNR_Position_R1/1 -> Terminator7/1
  in_IN_NodeDNR.DNR_Position.DNR_Position_N/1 -> Terminator6/1
  in_IN_NodeDNR.DNR_Position.DNR_Position_DM/1 -> Terminator5/1
  in_IN_NodeDNR.DNR_Position.DNR_Position_D7/1 -> Terminator4/1
  in_IN_NodeDNR.DNR_Position.DNR_Position_D4/1 -> Terminator3/1
  in_IN_NodeDNR.DNR_Position.DNR_Position_D1/1 -> Terminator2/1
  in_IN_NodeDNR.DNR_Position.DeviceState/1 -> Terminator1/1
  Constant3/1 -> out_OUT_LIN_01.ScheduleTable/1
  Constant2/1 -> out_OUT_LIN_01.LinNetworkRequest1/1
  Data Type Conversion1/1 -> out_OUT_Tester_1.BSG_STATUS.BatteryVoltage/1
  [u32Voltage] -> Data Type Conversion1/1
  Data Type Conversion/1 -> out_OUT_Tester_1.BSG_STATUS.Button_KL15/1
  [boIgnition] -> Data Type Conversion/1
  Constant1/1 -> out_OUT_Tester_1.BSG_STATUS.Voltage_Normal/1
  Constant/1 -> out_OUT_Tester_1.BSG_STATUS.Voltage_OV1/1, out_OUT_Tester_1.BSG_STATUS.Voltage_OV2/1, out_OUT_Tester_1.BSG_STATUS.Voltage_UV1/1, out_OUT_Tester_1.BSG_STATUS.Voltage_UV2/1
  Ground/1 -> bo_Out/1  "bo_Out"
  bo_In/1 -> Terminator/1

== system MBDS_Subsystems/SUB_SystemStates ==
  note: After POR, force model hold equal true during WakeUpForceHoldTime
  note: Wake-up Inputs
  u16_WakeUpForceHoldTime : Inport  OutDataTypeStr=uint16
  Ground : Ground  InitFcn=|
      | try
      |    MBDS_BlockCallback('Update', gcb);
      | end
      settings: MoveFcn=UpdateBlockSize(gcb);
  ModelHoldForceTrue : Stateflow chart  TreatAsAtomicUnit=on
      settings: CopyFcn=|
      | if(exist('MBDS_BlockCallback', 'file'))
      |    MBDS_BlockCallback('Copy', gcb);
      | end
  NOT : Subsystem  InitFcn=|  mask(NOT){MBDS_LibraryBlock=on, BitwiseMode=off, Inputs=1, UseBitMask=off, BitMask='A1', OutDataTypeStr=Inherit: Inherit via back propagation, MBDS_BlockVersion=08.20.02}
      | if(exist('MBDS_BlockCallback', 'file'))
      |    MBDS_BlockCallback('Update', gcb);
      | end
      mask prompts: MBDS_LibraryBlock "MBDS library block"; BitwiseMode "Use 'bitwise' mode"; Inputs "Number of input ports:"; UseBitMask "Use bit mask"; BitMask "Bit mask:"; OutDataTypeStr "Output data type:"; MBDS_BlockVersion "Version:"
      mask help: Logical or bitwise NOT operator. The input value is inverted. In bitwise mode all bits of the input signal are inverted.
      mask init: same as MBDS_Subsystems/SUB_DateTime/AND
      mask Help: eval(['open([workdir(''library_dir:''),''\Blockset\help\'',get_param(gcb,''MaskType''),''.html''])'])
      mask Callback BitwiseMode:
      | if(exist('MBDS_BlockCallback', 'file'))
      |    MBDS_BlockCallback('BitwiseMode', gcb);
      | end
      mask TypeOptions OutDataTypeStr: Inherit: Inherit via back propagation | int8 | uint8 | int16 | uint16 | int32 | uint32 | boolean
      mask Callback OutDataTypeStr:
      | % Adopt Value
      | if(exist('MBDS_BlockCallback', 'file'))
      |    MBDS_BlockCallback('OutDataTypeStr', gcb);
      | end
      mask DialogControl ParameterTabVar0 Prompt: Main
      mask DialogControl ParameterTabVar01 Prompt: Signal Attributes
      mask DialogControl ParameterTabVar012 Prompt: Version
      mask Display:
      | % Show icon or block text
      | disp('NOT')
  OR : Subsystem  InitFcn=|  mask(OR){MBDS_LibraryBlock=on, BitwiseMode=off, Inputs=8, UseBitMask=off, BitMask='A1', OutDataTypeStr=Inherit: Inherit via back propagation, MBDS_BlockVersion=08.20.02}
      | if(exist('MBDS_BlockCallback', 'file'))
      |    MBDS_BlockCallback('Update', gcb);
      | end
      mask prompts: MBDS_LibraryBlock "MBDS library block"; BitwiseMode "Use 'bitwise' mode"; Inputs "Number of input ports:"; UseBitMask "Use bit mask"; BitMask "Bit mask:"; OutDataTypeStr "Output data type:"; MBDS_BlockVersion "Version:"
      mask help: Logical or bitwise OR operator. For multiple inputs, operators are applied across the inputs. For a single input, operators are applied across the input vector. In bitwise mode a bit mask can be applied onto single input signals.
      mask init: same as MBDS_Subsystems/SUB_DateTime/AND
      mask Help: eval(['open([workdir(''library_dir:''),''\Blockset\help\'',get_param(gcb,''MaskType''),''.html''])'])
      mask Callback BitwiseMode:
      | if(exist('MBDS_BlockCallback', 'file'))
      |    MBDS_BlockCallback('BitwiseMode', gcb);
      | end
      mask Callback Inputs:
      | if(exist('MBDS_BlockCallback', 'file'))
      |    MBDS_BlockCallback('Inputs', gcb);
      | end
      mask Callback UseBitMask:
      | if(exist('MBDS_BlockCallback', 'file'))
      |    MBDS_BlockCallback('UseBitMask', gcb);
      | end
      mask Callback BitMask:
      | if(exist('MBDS_BlockCallback', 'file'))
      |    MBDS_BlockCallback('BitMask', gcb);
      | end
      mask TypeOptions OutDataTypeStr: Inherit: Inherit via back propagation | int8 | uint8 | int16 | uint16 | int32 | uint32 | boolean
      mask Callback OutDataTypeStr:
      | % Adopt Value
      | if(exist('MBDS_BlockCallback', 'file'))
      |    MBDS_BlockCallback('OutDataTypeStr', gcb);
      | end
      mask DialogControl ParameterTabVar0 Prompt: Main
      mask DialogControl ParameterTabVar01 Prompt: Signal Attributes
      mask DialogControl ParameterTabVar012 Prompt: Version
      mask Display:
      | % Show icon or block text
      | if(UseBitMask)
      |    if(isnumeric(BitMask))
      |       BitMaskString = ['0x',dec2hex(floor(BitMask))];
      |    elseif(ischar(BitMask))
      |       BitMaskString = ['0x',upper(BitMask)];
      |    else
      |       BitMaskString = '???';
      |    end
      |    disp(sprintf(['OR\n', BitMaskString]))
      | else
      |    disp('OR')
      | end
  in_INOUT_RAMDevice.boSystemWake : KIBES_Signal/KIBES_Signal  MBDS_LibraryBlock=on  DatabaseKey=3  SignalName=INOUT_RAMDevice.boSystemWake  SymbolName=INOUT_RAMDevice_boSystemWake_000003  DataType=boolean  Init=0  Slope=1  Bias=0  DataSize=1  fpDataType=boolean  BlockIOType=Inport  DeviceType=0
  in_IN_DigitalInputs.IN_DIG_02 : KIBES_Signal/KIBES_Signal  MBDS_LibraryBlock=on  DatabaseKey=35  SignalName=IN_DigitalInputs.IN_DIG_02  SymbolName=IN_DigitalInputs_IN_DIG_02_000035  DataType=boolean  Init=0  Slope=1  Bias=0  DataSize=1  fpDataType=boolean  BlockIOType=Inport  DeviceType=0
  in_IN_DigitalInputs.IN_DIG_10 : KIBES_Signal/KIBES_Signal  MBDS_LibraryBlock=on  DatabaseKey=96  SignalName=IN_DigitalInputs.IN_DIG_10  SymbolName=IN_DigitalInputs_IN_DIG_10_000096  DataType=boolean  Init=0  Slope=1  Bias=0  DataSize=1  fpDataType=boolean  BlockIOType=Inport  DeviceType=0
  in_IN_DigitalInputs.IN_DIG_17 : KIBES_Signal/KIBES_Signal  MBDS_LibraryBlock=on  DatabaseKey=16  SignalName=IN_DigitalInputs.IN_DIG_17  SymbolName=IN_DigitalInputs_IN_DIG_17_000016  DataType=boolean  Init=0  Slope=1  Bias=0  DataSize=1  fpDataType=boolean  BlockIOType=Inport  DeviceType=0
  in_IN_DigitalInputs.IN_DIG_26 : KIBES_Signal/KIBES_Signal  MBDS_LibraryBlock=on  DatabaseKey=34  SignalName=IN_DigitalInputs.IN_DIG_26  SymbolName=IN_DigitalInputs_IN_DIG_26_000034  DataType=boolean  Init=0  Slope=1  Bias=0  DataSize=1  fpDataType=boolean  BlockIOType=Inport  DeviceType=0
  in_IN_DigitalInputs.IN_DIG_35 : KIBES_Signal/KIBES_Signal  MBDS_LibraryBlock=on  DatabaseKey=58  SignalName=IN_DigitalInputs.IN_DIG_35  SymbolName=IN_DigitalInputs_IN_DIG_35_000058  DataType=boolean  Init=0  Slope=1  Bias=0  DataSize=1  fpDataType=boolean  BlockIOType=Inport  DeviceType=0
  in_IN_DigitalInputs.IN_DIG_36 : KIBES_Signal/KIBES_Signal  MBDS_LibraryBlock=on  DatabaseKey=60  SignalName=IN_DigitalInputs.IN_DIG_36  SymbolName=IN_DigitalInputs_IN_DIG_36_000060  DataType=boolean  Init=0  Slope=1  Bias=0  DataSize=1  fpDataType=boolean  BlockIOType=Inport  DeviceType=0
  in_IN_DigitalInputs.IN_DIG_40 : KIBES_Signal/KIBES_Signal  MBDS_LibraryBlock=on  DatabaseKey=68  SignalName=IN_DigitalInputs.IN_DIG_40  SymbolName=IN_DigitalInputs_IN_DIG_40_000068  DataType=boolean  Init=0  Slope=1  Bias=0  DataSize=1  fpDataType=boolean  BlockIOType=Inport  DeviceType=0
  out_INOUT_RAMDevice.boSystemWake : KIBES_Signal/KIBES_Signal  MBDS_LibraryBlock=on  DatabaseKey=3  SignalName=INOUT_RAMDevice.boSystemWake  SymbolName=INOUT_RAMDevice_boSystemWake_000003  DataType=boolean  Init=0  Slope=1  Bias=0  DataSize=1  fpDataType=boolean  BlockIOType=Outport  DeviceType=0
  out_OUT_ModelControl.ModelHold : KIBES_Signal/KIBES_Signal  MBDS_LibraryBlock=on  DatabaseKey=1  SignalName=OUT_ModelControl.ModelHold  SymbolName=OUT_ModelControl_ModelHold_000001  DataType=boolean  Init=0  Slope=1  Bias=0  DataSize=1  fpDataType=boolean  BlockIOType=Outport  DeviceType=0
  bo_Out : Outport  OutDataTypeStr=boolean
  wires:
  Ground/1 -> bo_Out/1  "bo_Out"
  u16_WakeUpForceHoldTime/1 -> ModelHoldForceTrue/1(u16_WakeUpForceHoldTime)
  ModelHoldForceTrue/1(bo_ModelHold) -> OR/8(u8)
  OR/1(y) -> out_INOUT_RAMDevice.boSystemWake/1
  in_INOUT_RAMDevice.boSystemWake/1 -> out_OUT_ModelControl.ModelHold/1
  in_IN_DigitalInputs.IN_DIG_40/1 -> OR/7(u7)
  in_IN_DigitalInputs.IN_DIG_36/1 -> OR/6(u6)
  in_IN_DigitalInputs.IN_DIG_35/1 -> OR/5(u5)
  in_IN_DigitalInputs.IN_DIG_26/1 -> OR/4(u4)
  in_IN_DigitalInputs.IN_DIG_17/1 -> NOT/1(u1)
  in_IN_DigitalInputs.IN_DIG_10/1 -> OR/2(u2)
  in_IN_DigitalInputs.IN_DIG_02/1 -> OR/1(u1)
  NOT/1(y) -> OR/3(u3)

== system MBDS_Subsystems/SUB_TsuControl ==
  bo_In : Inport  OutDataTypeStr=boolean
  Constant : Constant  InitFcn=|  Value=true  OutDataTypeStr=boolean
      | if(exist('MBDS_BlockCallback', 'file'))
      |    MBDS_BlockCallback('Update', gcb);  
      | end
  Constant1 : Constant  InitFcn=|  Value=0  OutDataTypeStr=uint8
      | if(exist('MBDS_BlockCallback', 'file'))
      |    MBDS_BlockCallback('Update', gcb);  
      | end
  Ground : Ground  InitFcn=|
      | try
      |    MBDS_BlockCallback('Update', gcb);
      | end
      settings: MoveFcn=UpdateBlockSize(gcb);
  Terminator : Terminator
      settings: MoveFcn=UpdateBlockSize(gcb);
      settings: InitFcn=|
      | try
      |    MBDS_BlockCallback('Update', gcb);
      | end
  in_DIAG_TSUD.ShaftSpeed_DIAG : KIBES_Signal/KIBES_Signal  MBDS_LibraryBlock=on  DatabaseKey=1301  SignalName=DIAG_TSUD.ShaftSpeed_DIAG  SymbolName=DIAG_TSUD_ShaftSpeed_DIAG_001301  DataType=uint16  Init=1  Slope=1  Bias=0  DataSize=1  fpDataType=uint16  BlockIOType=Inport  DeviceType=0
  in_DIAG_TSUD.VehicleSpeed_DIAG : KIBES_Signal/KIBES_Signal  MBDS_LibraryBlock=on  DatabaseKey=1303  SignalName=DIAG_TSUD.VehicleSpeed_DIAG  SymbolName=DIAG_TSUD_VehicleSpeed_DIAG_001303  DataType=uint16  Init=1  Slope=1  Bias=0  DataSize=1  fpDataType=uint16  BlockIOType=Inport  DeviceType=0
  in_INOUT_RAMDevice.boSystemWake : KIBES_Signal/KIBES_Signal  MBDS_LibraryBlock=on  DatabaseKey=3  SignalName=INOUT_RAMDevice.boSystemWake  SymbolName=INOUT_RAMDevice_boSystemWake_000003  DataType=boolean  Init=0  Slope=1  Bias=0  DataSize=1  fpDataType=boolean  BlockIOType=Inport  DeviceType=0
  in_IN_TSUD.ShaftSpeed : KIBES_Signal/KIBES_Signal  MBDS_LibraryBlock=on  DatabaseKey=1300  SignalName=IN_TSUD.ShaftSpeed  SymbolName=IN_TSUD_ShaftSpeed_001300  DataType=uint16  Init=0  Slope=1  Bias=0  DataSize=1  fpDataType=uint16  BlockIOType=Inport  DeviceType=0
  in_IN_TSUD.VehicleSpeed : KIBES_Signal/KIBES_Signal  MBDS_LibraryBlock=on  DatabaseKey=1302  SignalName=IN_TSUD.VehicleSpeed  SymbolName=IN_TSUD_VehicleSpeed_001302  DataType=uint16  Init=0  Slope=1  Bias=0  DataSize=1  fpDataType=uint16  BlockIOType=Inport  DeviceType=0
  out_OUT_PCAN.Tx_Tsu.TSU_Sts.MessageEnable : KIBES_Signal/KIBES_Signal  MBDS_LibraryBlock=on  DatabaseKey=1805  SignalName=OUT_PCAN.Tx_Tsu.TSU_Sts.MessageEnable  SymbolName=OUT_PCAN_Tx_Tsu_TSU_Sts_MessageEnable_001805  DataType=boolean  Init=0  Slope=1  Bias=0  DataSize=1  fpDataType=boolean  BlockIOType=Outport  DeviceType=0
  out_OUT_PCAN.Tx_Tsu.TSU_Sts.Speed_Shaft : KIBES_Signal/KIBES_Signal  MBDS_LibraryBlock=on  DatabaseKey=1804  SignalName=OUT_PCAN.Tx_Tsu.TSU_Sts.Speed_Shaft  SymbolName=OUT_PCAN_Tx_Tsu_TSU_Sts_Speed_Shaft_001804  DataType=uint16  Init=0  Slope=1  Bias=0  DataSize=1  fpDataType=uint16  BlockIOType=Outport  DeviceType=0
  out_OUT_PCAN.Tx_Tsu.TSU_Sts.Speed_Shaft_DIAG : KIBES_Signal/KIBES_Signal  MBDS_LibraryBlock=on  DatabaseKey=1803  SignalName=OUT_PCAN.Tx_Tsu.TSU_Sts.Speed_Shaft_DIAG  SymbolName=OUT_PCAN_Tx_Tsu_TSU_Sts_Speed_Shaft_DIAG_001803  DataType=uint16  Init=0  Slope=1  Bias=0  DataSize=1  fpDataType=uint16  BlockIOType=Outport  DeviceType=0
  out_OUT_PCAN.Tx_Tsu.TSU_Sts.Speed_Vehicle : KIBES_Signal/KIBES_Signal  MBDS_LibraryBlock=on  DatabaseKey=1802  SignalName=OUT_PCAN.Tx_Tsu.TSU_Sts.Speed_Vehicle  SymbolName=OUT_PCAN_Tx_Tsu_TSU_Sts_Speed_Vehicle_001802  DataType=uint16  Init=0  Slope=1  Bias=0  DataSize=1  fpDataType=uint16  BlockIOType=Outport  DeviceType=0
  out_OUT_PCAN.Tx_Tsu.TSU_Sts.Speed_Vehicle_DIAG : KIBES_Signal/KIBES_Signal  MBDS_LibraryBlock=on  DatabaseKey=1801  SignalName=OUT_PCAN.Tx_Tsu.TSU_Sts.Speed_Vehicle_DIAG  SymbolName=OUT_PCAN_Tx_Tsu_TSU_Sts_Speed_Vehicle_DIAG_001801  DataType=uint16  Init=0  Slope=1  Bias=0  DataSize=1  fpDataType=uint16  BlockIOType=Outport  DeviceType=0
  out_OUT_TSUD.DeviceEnable : KIBES_Signal/KIBES_Signal  MBDS_LibraryBlock=on  DatabaseKey=1297  SignalName=OUT_TSUD.DeviceEnable  SymbolName=OUT_TSUD_DeviceEnable_001297  DataType=boolean  Init=0  Slope=1  Bias=0  DataSize=1  fpDataType=boolean  BlockIOType=Outport  DeviceType=0
  out_OUT_TSUD.SetDiagWriteOdoResponse : KIBES_Signal/KIBES_Signal  MBDS_LibraryBlock=on  DatabaseKey=1304  SignalName=OUT_TSUD.SetDiagWriteOdoResponse  SymbolName=OUT_TSUD_SetDiagWriteOdoResponse_001304  DataType=uint8  Init=0  Slope=1  Bias=0  DataSize=1  fpDataType=uint8  BlockIOType=Outport  DeviceType=0
  bo_Out : Outport  OutDataTypeStr=boolean
  wires:
  Constant1/1 -> out_OUT_TSUD.SetDiagWriteOdoResponse/1
  Constant/1 -> out_OUT_TSUD.DeviceEnable/1
  in_DIAG_TSUD.VehicleSpeed_DIAG/1 -> out_OUT_PCAN.Tx_Tsu.TSU_Sts.Speed_Vehicle_DIAG/1
  in_IN_TSUD.VehicleSpeed/1 -> out_OUT_PCAN.Tx_Tsu.TSU_Sts.Speed_Vehicle/1
  in_DIAG_TSUD.ShaftSpeed_DIAG/1 -> out_OUT_PCAN.Tx_Tsu.TSU_Sts.Speed_Shaft_DIAG/1
  in_IN_TSUD.ShaftSpeed/1 -> out_OUT_PCAN.Tx_Tsu.TSU_Sts.Speed_Shaft/1
  in_INOUT_RAMDevice.boSystemWake/1 -> out_OUT_PCAN.Tx_Tsu.TSU_Sts.MessageEnable/1
  Ground/1 -> bo_Out/1  "bo_Out"
  bo_In/1 -> Terminator/1

== system MBDS_Subsystems/SUB_DateTime/AND ==
  note: AND
  u1 : Inport  OutDataTypeStr=boolean
  u2 : Inport  Port=2  OutDataTypeStr=boolean
  DataType : DataTypeConversion  OutDataTypeStr=boolean
  Operator : Logic  AllPortsSameDT=off  OutDataTypeStr=boolean
  y : Outport
  wires:
  DataType/1 -> y/1
  u2/1 -> Operator/2
  u1/1 -> Operator/1
  Operator/1 -> DataType/1

== system MBDS_Subsystems/SUB_DateTime/EQ ==
  note: EQ
  u1 : Inport
  u2 : Inport  Port=2
  Operator : RelationalOperator  Operator===  OutDataTypeStr=boolean  RndMeth=Nearest  InputSameDT=on
  y : Outport
  wires:
  u2/1 -> Operator/2
  u1/1 -> Operator/1
  Operator/1 -> y/1
